simulink model "test1_external_code"  (R2016a)
settings: Solver=FixedStepAuto  StartTime=0.0  StopTime=55  FixedStep=0.02  MaxStep=0.001  RelTol=1e-3
undefined symbols (not defined in the file or in its folder): get, hot
libraries: tinbot x3, dspsnks4 x1
(part 2 of 2)

== stateflow chart test1_external_code/Chart ==
  state Start
  (default) -> Start
  Start -> Start : {
      | 	update_sensors(&controller, proximity, ir);
      | 	motor_left = controller.motor_left;
      | 	motor_right = controller.motor_right;
      | }
  data: proximity input size=8; ir input size=6; motor_left output double; motor_right output double; controller local Bus: Controller
